simulink model "s_6dof2016a"  (R2016a)
settings: Solver=VariableStepAuto  SolverMode=SingleTasking  StartTime=0.0  StopTime=90  RelTol=1e-3
(part 1 of 2)
settings Model: Creator=Admin  LastModifiedBy=HP
settings DebuggingCC: SFUnexpectedBacktrackingDiag=error  SFNoUnconditionalDefaultTransitionDiag=error
settings GRTTargetCC: TargetLangStandard=C99 (ISO)  GeneratePreprocessorConditionals=Use local settings
settings ConfigComp: CovMetricSettings=dwe  CovHtmlReporting=off  CovSaveCumulativeToWorkspaceVar=off  CovSaveSingleToWorkspaceVar=off  CovExternalEMLEnable=on

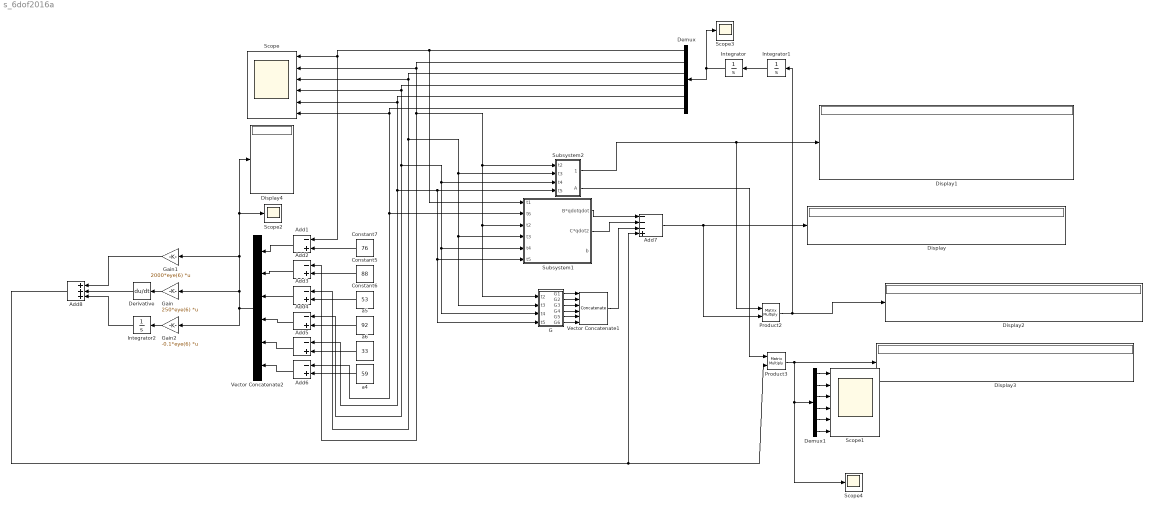
== system s_6dof2016a ==
  Add{1..6} (6 alike) : Sum  Inputs=-+
  Add7 : Sum  Inputs=---+
  Add8 : Sum  Inputs=+++
  Constant5 : Constant  Value=88
  Constant6 : Constant  Value=53
  Constant7 : Constant  Value=76
  Demux : Demux  Outputs=6
  Demux1 : Demux  Outputs=6
  Derivative : Derivative
  Display{,1..4} (5 alike) : Display
  G : Subsystem
  Gain : Gain  Gain=250*eye(6)  Multiplication=Matrix(K*u)
  Gain1 : Gain  Gain=2000*eye(6)  Multiplication=Matrix(K*u)
  Gain2 : Gain  Gain=-0.1*eye(6)  Multiplication=Matrix(K*u)
  Integrator : Integrator
  Integrator1 : Integrator
  Integrator2 : Integrator
  Product2 : Product  Multiplication=Matrix(*)
  Product3 : Product  Multiplication=Matrix(*)
  Scope : Scope  NumInputPorts=6
  Scope1 : Scope  NumInputPorts=6
  Scope2 : Scope
  Scope3 : Scope
  Scope4 : Scope
  Subsystem1 : Subsystem
  Subsystem2 : Subsystem
  Vector Concatenate1 : Concatenate  NumInputs=6  Mode=Multidimensional array
  Vector Concatenate2 : Concatenate  NumInputs=6  Mode=Multidimensional array
  a4 : Constant  Value=59
  a5 : Constant  Value=92
  a6 : Constant  Value=33
  wires:
  Demux/4 -> Scope/4, Add4/1, G/3(t4), Subsystem1/5("t4 "), Subsystem2/3(t4)
  Demux/5 -> Scope/5, Add5/1, G/4(t5), Subsystem1/6(t5), Subsystem2/4(t5)
  Demux/2 -> Scope/2, Add2/1, G/1(t2), Subsystem1/3(t2), Subsystem2/1(t2)
  Demux/3 -> Scope/3, G/2(t3), Subsystem1/4(t3), Subsystem2/2(t3), Add3/1
  Demux/1 -> Scope/1, Add1/1, Subsystem1/1(t1)
  Demux/6 -> Scope/6, Subsystem1/2(t6), Add6/1
  Constant7/1 -> Add1/2
  Constant5/1 -> Add2/2
  Constant6/1 -> Add3/2
  a5/1 -> Add4/2
  a6/1 -> Add5/2
  a4/1 -> Add6/2
  Subsystem1/1(B*qdotqdot) -> Add7/1
  Subsystem1/2(C*qdot2) -> Add7/2
  G/1(G1) -> Vector Concatenate1/1
  G/2(G2) -> Vector Concatenate1/2
  G/3(G3) -> Vector Concatenate1/3
  G/6(G6) -> Vector Concatenate1/6
  G/4(G4) -> Vector Concatenate1/4
  G/5(G5) -> Vector Concatenate1/5
  Vector Concatenate1/1 -> Add7/3
  Add7/1 -> Product2/2, Display/1
  Subsystem2/1(A inv) -> Product2/1, Display1/1
  Add2/1 -> Vector Concatenate2/2
  Add1/1 -> Vector Concatenate2/1
  Add3/1 -> Vector Concatenate2/3
  Add4/1 -> Vector Concatenate2/4
  Add5/1 -> Vector Concatenate2/5
  Add6/1 -> Vector Concatenate2/6
  Product2/1 -> Integrator1/1, Display2/1
  Integrator1/1 -> Integrator/1
  Integrator/1 -> Scope3/1, Demux/1
  Product3/1 -> Scope4/1, Demux1/1, Display3/1
  Subsystem2/2("A ") -> Product3/1
  Demux1/1 -> Scope1/1
  Demux1/2 -> Scope1/2
  Demux1/3 -> Scope1/3
  Demux1/4 -> Scope1/4
  Demux1/5 -> Scope1/5
  Demux1/6 -> Scope1/6
  Vector Concatenate2/1 -> Display4/1, Scope2/1, Gain1/1, Gain/1, Gain2/1
  Gain/1 -> Derivative/1
  Gain2/1 -> Integrator2/1
  Gain1/1 -> Add8/1
  Add8/1 -> Product3/2, Add7/4
  Derivative/1 -> Add8/2
  Integrator2/1 -> Add8/3

== system s_6dof2016a/G ==
  t2 : Inport
  t3 : Inport  Port=2
  t4 : Inport  Port=3
  t5 : Inport  Port=4
  g1 : Constant  Value=0
  g2 : Subsystem
  g3 : Subsystem
  g4 : Subsystem
  g5 : Subsystem
  g6 : Constant  Value=0
  G1 : Outport
  G2 : Outport  Port=2
  G3 : Outport  Port=3
  G4 : Outport  Port=4
  G5 : Outport  Port=5
  G6 : Outport  Port=6
  wires:
  t5/1 -> g5/2(t5), g4/2(t5)
  g3/1(g3) -> G3/1
  g5/1(g5) -> G5/1
  t3/1 -> g5/4(t3), g4/4(t3), g3/2(t3), g2/2(t3)
  t4/1 -> g5/1(t4), g4/1(t4)
  g2/1(g2) -> G2/1
  t2/1 -> g5/3(t2), g4/3(t2), g3/1(t2), g2/1(t2)
  g1/1 -> G1/1
  g4/1(g4) -> G4/1
  g6/1 -> G6/1

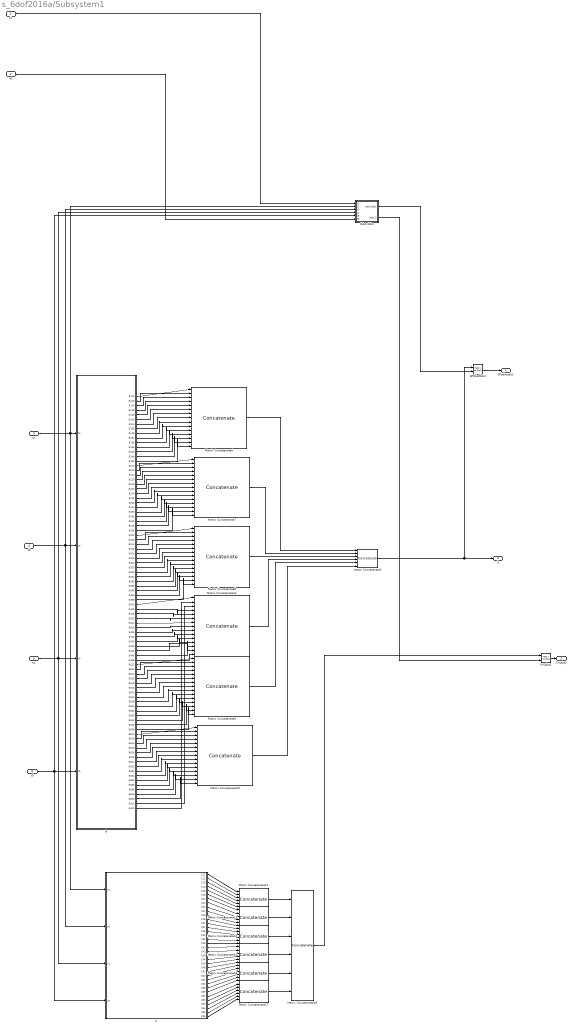
== system s_6dof2016a/Subsystem1 ==
  t1 : Inport
  t6 : Inport  Port=2
  t2 : Inport  Port=3
  t3 : Inport  Port=4
  "t4 " : Inport  Port=5
  t5 : Inport  Port=6
  B : Subsystem
  B*QdotQdot : Product  Multiplication=Matrix(*)
  C : Subsystem
  C*Qdot2 : Product  Multiplication=Matrix(*)
  Matrix Concatenate{6..11} (6 alike) : Concatenate  NumInputs=15  Mode=Multidimensional array  ConcatenateDimension=2
  Matrix Concatenate{12..17} (6 alike) : Concatenate  NumInputs=6  Mode=Multidimensional array  ConcatenateDimension=2
  Matrix Concatenate18 : Concatenate  NumInputs=6  Mode=Multidimensional array
  Qdot,Qdot : Subsystem
  Vector Concatenate1 : Concatenate  NumInputs=6  Mode=Multidimensional array
  B*qdotqdot : Outport
  C*qdot2 : Outport  Port=2
  "b " : Outport  Port=3
  wires:
  C/29(C55) -> Matrix Concatenate16/5
  C/31(C61) -> Matrix Concatenate17/1
  B/15(B156) -> Matrix Concatenate6/15
  C/25(C51) -> Matrix Concatenate16/1
  B/47(B415) -> Matrix Concatenate11/4
  C/24(C46) -> Matrix Concatenate15/6
  B/22(B224) -> Matrix Concatenate7/7
  "t4 "/1 -> C/3(t4), Qdot,Qdot/4(t4), B/3(t4)
  B/36(B323) -> Matrix Concatenate8/6
  C/30(C56) -> Matrix Concatenate16/6
  B*QdotQdot/1 -> B*qdotqdot/1
  B/37(B324) -> Matrix Concatenate8/7
  t5/1 -> Qdot,Qdot/5(t5), C/4(t5), B/4(t5)
  B/17(B213) -> Matrix Concatenate7/2
  C/10(C24) -> Matrix Concatenate13/4
  C/28(C54) -> Matrix Concatenate16/4
  B/10(B134) -> Matrix Concatenate6/10
  C/33(C63) -> Matrix Concatenate17/3
  Qdot,Qdot/2(qdot,2) -> C*Qdot2/2
  B/26(B235) -> Matrix Concatenate7/11
  C/7(C21) -> Matrix Concatenate13/1
  C/20(C42) -> Matrix Concatenate15/2
  B/67(B526) -> Matrix Concatenate9/9
  C/23(C45) -> Matrix Concatenate15/5
  B/7(B124) -> Matrix Concatenate6/7
  B/84(B635) -> Matrix Concatenate10/11
  C/11(C25) -> Matrix Concatenate13/5
  B/14(B146) -> Matrix Concatenate6/14
  C/19(C41) -> Matrix Concatenate15/1
  C/26(C52) -> Matrix Concatenate16/2
  B/45(B356) -> Matrix Concatenate8/15
  B/24(B226) -> Matrix Concatenate7/9
  C/35(C65) -> Matrix Concatenate17/5
  B/59(B512) -> Matrix Concatenate9/1
  C/6(C16) -> Matrix Concatenate12/6
  B/23(B225) -> Matrix Concatenate7/8
  C/21(C43) -> Matrix Concatenate15/3
  B/13(B145) -> Matrix Concatenate6/13
  C/36(C66) -> Matrix Concatenate17/6
  t2/1 -> Qdot,Qdot/2(t2), C/1(t2), B/1(t2)
  C/32(C62) -> Matrix Concatenate17/2
  B/63(B516) -> Matrix Concatenate9/5
  t3/1 -> Qdot,Qdot/3(t3), C/2(t3), B/2(t3)
  Matrix Concatenate12/1 -> Matrix Concatenate18/1
  B/65(B524) -> Matrix Concatenate9/7
  C/8(C22) -> Matrix Concatenate13/2
  B/6(B123) -> Matrix Concatenate6/6
  C/13(C31) -> Matrix Concatenate14/1
  B/61(B514) -> Matrix Concatenate9/3
  Matrix Concatenate18/1 -> C*Qdot2/1
  C/9(C23) -> Matrix Concatenate13/3
  C/12(C26) -> Matrix Concatenate13/6
  B/78(B616) -> Matrix Concatenate10/5
  B/4(B115) -> Matrix Concatenate6/4
  B/35(B316) -> Matrix Concatenate8/5
  C/16(C34) -> Matrix Concatenate14/4
  C/14(C32) -> Matrix Concatenate14/2
  B/66(B525) -> Matrix Concatenate9/8
  C/18(C36) -> Matrix Concatenate14/6
  B/32(B313) -> Matrix Concatenate8/2
  C/17(C35) -> Matrix Concatenate14/5
  B/2(B113) -> Matrix Concatenate6/2
  B/25(B234) -> Matrix Concatenate7/10
  B/11(B135) -> Matrix Concatenate6/11
  B/18(B214) -> Matrix Concatenate7/3
  B/77(B615) -> Matrix Concatenate10/4
  B/5(B116) -> Matrix Concatenate6/5
  B/64(B523) -> Matrix Concatenate9/6
  t1/1 -> Qdot,Qdot/1(t1)
  B/3(B114) -> Matrix Concatenate6/3
  B/27(B236) -> Matrix Concatenate7/12
  B/28(B245) -> Matrix Concatenate7/13
  B/30(B256) -> Matrix Concatenate7/15
  B/51(B425) -> Matrix Concatenate11/8
  B/40(B334) -> Matrix Concatenate8/10
  B/60(B513) -> Matrix Concatenate9/2
  B/70(B536) -> Matrix Concatenate9/12
  B/74(B612) -> Matrix Concatenate10/1
  B/75(B613) -> Matrix Concatenate10/2
  B/79(B623) -> Matrix Concatenate10/6
  B/80(B624) -> Matrix Concatenate10/7
  B/21(B223) -> Matrix Concatenate7/6
  t6/1 -> Qdot,Qdot/6(t6)
  B/31(B312) -> Matrix Concatenate8/1
  B/42(B336) -> Matrix Concatenate8/12
  B/81(B625) -> Matrix Concatenate10/8
  B/9(B126) -> Matrix Concatenate6/9
  B/68(B534) -> Matrix Concatenate9/10
  B/29(B246) -> Matrix Concatenate7/14
  B/38(B325) -> Matrix Concatenate8/8
  B/52(B426) -> Matrix Concatenate11/9
  B/82(B626) -> Matrix Concatenate10/9
  B/86(B645) -> Matrix Concatenate10/13
  B/43(B345) -> Matrix Concatenate8/13
  B/71(B545) -> Matrix Concatenate9/13
  B/87(B646) -> Matrix Concatenate10/14
  B/46(B412) -> Matrix Concatenate11/1
  B/83(B634) -> Matrix Concatenate10/10
  B/89(B414) -> Matrix Concatenate11/3
  B/69(B535) -> Matrix Concatenate9/11
  B/33(B314) -> Matrix Concatenate8/3
  B/20(B216) -> Matrix Concatenate7/5
  B/90(B413) -> Matrix Concatenate11/2
  B/76(B614) -> Matrix Concatenate10/3
  B/50(B424) -> Matrix Concatenate11/7
  B/19(B215) -> Matrix Concatenate7/4
  B/62(B515) -> Matrix Concatenate9/4
  B/57(B446) -> Matrix Concatenate11/14
  Matrix Concatenate7/1 -> Vector Concatenate1/2
  B/48(B416) -> Matrix Concatenate11/5
  B/34(B315) -> Matrix Concatenate8/4
  B/1(B112) -> Matrix Concatenate6/1
  B/53(B434) -> Matrix Concatenate11/10
  B/54(B435) -> Matrix Concatenate11/11
  Matrix Concatenate14/1 -> Matrix Concatenate18/3
  B/73(B556) -> Matrix Concatenate9/15
  Matrix Concatenate8/1 -> Vector Concatenate1/3
  C/1(C11) -> Matrix Concatenate12/1
  B/85(B636) -> Matrix Concatenate10/12
  Matrix Concatenate9/1 -> Vector Concatenate1/5
  B/39(B326) -> Matrix Concatenate8/9
  B/49(B423) -> Matrix Concatenate11/6
  Matrix Concatenate11/1 -> Vector Concatenate1/4
  B/55(B436) -> Matrix Concatenate11/12
  B/41(B335) -> Matrix Concatenate8/11
  B/16(B212) -> Matrix Concatenate7/1
  Matrix Concatenate10/1 -> Vector Concatenate1/6
  C/34(C64) -> Matrix Concatenate17/4
  B/56(B445) -> Matrix Concatenate11/13
  B/44(B346) -> Matrix Concatenate8/14
  B/88(B656) -> Matrix Concatenate10/15
  Qdot,Qdot/1(qdot,qdot) -> B*QdotQdot/2
  B/72(B546) -> Matrix Concatenate9/14
  B/12(B136) -> Matrix Concatenate6/12
  B/58(B456) -> Matrix Concatenate11/15
  Matrix Concatenate6/1 -> Vector Concatenate1/1
  B/8(B125) -> Matrix Concatenate6/8
  Vector Concatenate1/1 -> "b "/1, B*QdotQdot/1
  C/22(C44) -> Matrix Concatenate15/4
  C/15(C33) -> Matrix Concatenate14/3
  C/27(C53) -> Matrix Concatenate16/3
  Matrix Concatenate17/1 -> Matrix Concatenate18/6
  Matrix Concatenate16/1 -> Matrix Concatenate18/5
  Matrix Concatenate13/1 -> Matrix Concatenate18/2
  Matrix Concatenate15/1 -> Matrix Concatenate18/4
  C/3(C13) -> Matrix Concatenate12/3
  C/2(C12) -> Matrix Concatenate12/2
  C/4(C14) -> Matrix Concatenate12/4
  C/5(C15) -> Matrix Concatenate12/5
  C*Qdot2/1 -> C*qdot2/1

== system s_6dof2016a/Subsystem2 ==
  t2 : Inport
  t3 : Inport  Port=2
  t4 : Inport  Port=3
  t5 : Inport  Port=4
  Divide : Product  Inputs=/  Multiplication=Matrix(*)
  Matrix Concatenate{,1..5} (6 alike) : Concatenate  NumInputs=6  Mode=Multidimensional array  ConcatenateDimension=2
  Subsystem : Subsystem
  Vector Concatenate : Concatenate  NumInputs=6  Mode=Multidimensional array
  A inv : Outport
  "A " : Outport  Port=2
  wires:
  Subsystem/5(A15) -> Matrix Concatenate/5
  Subsystem/13(A31) -> Matrix Concatenate2/1
  Subsystem/12(A26) -> Matrix Concatenate1/6
  Subsystem/36(A66) -> Matrix Concatenate5/6
  Subsystem/1(A11) -> Matrix Concatenate/1
  Subsystem/24(A46) -> Matrix Concatenate3/6
  Subsystem/3(A13) -> Matrix Concatenate/3
  Subsystem/2(A12) -> Matrix Concatenate/2
  Subsystem/26(A52) -> Matrix Concatenate4/2
  Subsystem/28(A54) -> Matrix Concatenate4/4
  t5/1 -> Subsystem/4("t5 ")
  Subsystem/10(A24) -> Matrix Concatenate1/4
  Subsystem/9(A23) -> Matrix Concatenate1/3
  Subsystem/15(A33) -> Matrix Concatenate2/3
  Subsystem/11(A25) -> Matrix Concatenate1/5
  Subsystem/34(A64) -> Matrix Concatenate5/4
  Subsystem/18(A36) -> Matrix Concatenate2/6
  Matrix Concatenate4/1 -> Vector Concatenate/5
  Subsystem/19(A41) -> Matrix Concatenate3/1
  Subsystem/20(A42) -> Matrix Concatenate3/2
  Subsystem/23(A45) -> Matrix Concatenate3/5
  Subsystem/29(A55) -> Matrix Concatenate4/5
  Subsystem/30(A56) -> Matrix Concatenate4/6
  Subsystem/7(A21) -> Matrix Concatenate1/1
  t2/1 -> Subsystem/1(t2)
  Subsystem/33(A63) -> Matrix Concatenate5/3
  Subsystem/35(A65) -> Matrix Concatenate5/5
  Matrix Concatenate/1 -> Vector Concatenate/1
  Matrix Concatenate1/1 -> Vector Concatenate/2
  Matrix Concatenate2/1 -> Vector Concatenate/3
  Subsystem/21(A43) -> Matrix Concatenate3/3
  Subsystem/22(A44) -> Matrix Concatenate3/4
  Subsystem/25(A51) -> Matrix Concatenate4/1
  Subsystem/8(A22) -> Matrix Concatenate1/2
  Subsystem/4(A14) -> Matrix Concatenate/4
  Subsystem/6(A16) -> Matrix Concatenate/6
  Subsystem/31(A61) -> Matrix Concatenate5/1
  Subsystem/27(A53) -> Matrix Concatenate4/3
  Subsystem/17(A35) -> Matrix Concatenate2/5
  Matrix Concatenate5/1 -> Vector Concatenate/6
  Subsystem/14(A32) -> Matrix Concatenate2/2
  Subsystem/32(A62) -> Matrix Concatenate5/2
  t4/1 -> Subsystem/3(t4)
  Subsystem/16(A34) -> Matrix Concatenate2/4
  Matrix Concatenate3/1 -> Vector Concatenate/4
  t3/1 -> Subsystem/2(t3)
  Vector Concatenate/1 -> "A "/1, Divide/1
  Divide/1 -> A inv/1

== system s_6dof2016a/G/g2 ==
  t2 : Inport
  t3 : Inport  Port=2
  Add1 : Sum
  Add2 : Sum  Inputs=+++
  Product2 : Product
  Product3 : Product
  Product4 : Product
  Trigonometric Function1 : Trigonometry  Operator=cos
  Trigonometric Function4 : Trigonometry
  Trigonometric Function6 : Trigonometry
  c : Constant  Value=-37.2
  c2 : Constant  Value=-8.4
  c3 : Constant  Value=1.02
  g2 : Outport
  wires:
  c2/1 -> Product3/1
  t2/1 -> Trigonometric Function6/1, Add1/1, Trigonometric Function1/1
  Product4/1 -> Add2/3
  Product2/1 -> Add2/1
  Trigonometric Function6/1 -> Product4/2
  c3/1 -> Product4/1
  Add1/1 -> Trigonometric Function4/1
  Add2/1 -> g2/1
  Trigonometric Function4/1 -> Product3/2
  Product3/1 -> Add2/2
  Trigonometric Function1/1 -> Product2/2
  c/1 -> Product2/1
  t3/1 -> Add1/2

== system s_6dof2016a/G/g3 ==
  t2 : Inport
  t3 : Inport  Port=2
  Add1 : Sum
  Add2 : Sum
  Product2 : Product
  Product3 : Product
  Trigonometric Function1 : Trigonometry
  Trigonometric Function4 : Trigonometry  Operator=cos
  c2 : Constant  Value=-8.4
  c3 : Constant  Value=0.25
  g3 : Outport
  wires:
  Product2/1 -> Add2/1
  Trigonometric Function1/1 -> Product2/2
  Add1/1 -> Trigonometric Function4/1, Trigonometric Function1/1
  c2/1 -> Product2/1
  Product3/1 -> Add2/2
  t3/1 -> Add1/2
  c3/1 -> Product3/1
  t2/1 -> Add1/1
  Trigonometric Function4/1 -> Product3/2
  Add2/1 -> g3/1

== system s_6dof2016a/G/g4 ==
  t4 : Inport
  t5 : Inport  Port=2
  t2 : Inport  Port=3
  t3 : Inport  Port=4
  Add1 : Sum
  Product2 : Product  Inputs=4
  Trigonometric Function1 : Trigonometry
  Trigonometric Function4 : Trigonometry
  Trigonometric Function6 : Trigonometry
  c2 : Constant  Value=0.028
  g4 : Outport
  wires:
  t4/1 -> Trigonometric Function4/1
  Trigonometric Function4/1 -> Product2/3
  Product2/1 -> g4/1
  c2/1 -> Product2/1
  t5/1 -> Trigonometric Function6/1
  t2/1 -> Add1/1
  Trigonometric Function1/1 -> Product2/2
  Add1/1 -> Trigonometric Function1/1
  Trigonometric Function6/1 -> Product2/4
  t3/1 -> Add1/2

== system s_6dof2016a/G/g5 ==
  t4 : Inport
  t5 : Inport  Port=2
  t2 : Inport  Port=3
  t3 : Inport  Port=4
  Add1 : Sum
  Add2 : Sum
  Product2 : Product
  Product3 : Product  Inputs=3
  Product4 : Product
  Trigonometric Function1 : Trigonometry  Operator=cos
  Trigonometric Function4 : Trigonometry
  Trigonometric Function6 : Trigonometry
  Trigonometric Function7 : Trigonometry  Operator=cos
  Trigonometric Function8 : Trigonometry  Operator=cos
  c2 : Constant  Value=-0.028
  g5 : Outport
  wires:
  Add1/1 -> Trigonometric Function6/1, Trigonometric Function1/1
  c2/1 -> Product4/1
  Trigonometric Function1/1 -> Product2/1
  t5/1 -> Trigonometric Function8/1, Trigonometric Function4/1
  Trigonometric Function7/1 -> Product3/2
  Trigonometric Function6/1 -> Product3/1
  Trigonometric Function8/1 -> Product3/3
  Trigonometric Function4/1 -> Product2/2
  t2/1 -> Add1/1
  Product2/1 -> Add2/1
  Add2/1 -> Product4/2
  Product3/1 -> Add2/2
  t3/1 -> Add1/2
  t4/1 -> Trigonometric Function7/1
  Product4/1 -> g5/1

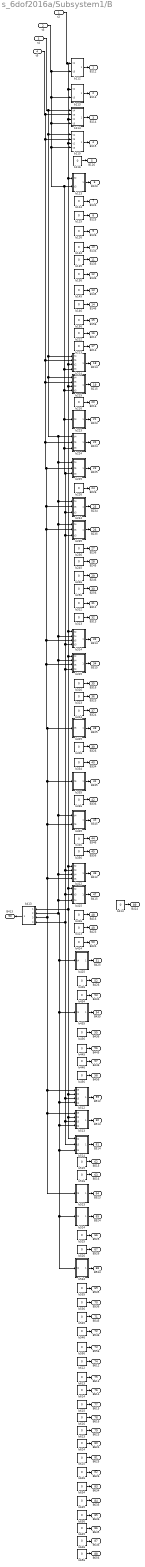
== system s_6dof2016a/Subsystem1/B ==
  t2 : Inport
  t3 : Inport  Port=2
  t4 : Inport  Port=3
  t5 : Inport  Port=4
  b112 : Subsystem
  b113 : Subsystem
  b114 : Subsystem
  b115 : Subsystem
  b{116,124..126,134..136,145..146,156,212..213,216,226,236,245..246,256,312..313,316,323..324,326,334,336,346,356,414,416,423..424,426,434,436,445..446,456,515..516,525..526,535..536,545..546,556,612..616,623..626,634..636,645..646,656} (62 alike) : Constant  Value=0
  b123 : Subsystem
  b214 : Subsystem
  b215 : Subsystem
  b223 : Subsystem
  b224 : Subsystem
  b225 : Subsystem
  b234 : Subsystem
  b235 : Subsystem
  b314 : Subsystem
  b315 : Subsystem
  b325 : Subsystem
  b335 : Subsystem
  b345 : Subsystem
  b412 : Subsystem
  b413 : Subsystem
  b415 : Subsystem
  b425 : Subsystem
  b435 : Subsystem
  b512 : Subsystem
  b513 : Subsystem
  b514 : Subsystem
  b523 : Subsystem
  b524 : Subsystem
  b534 : Subsystem
  B112 : Outport
  B113 : Outport  Port=2
  B114 : Outport  Port=3
  B115 : Outport  Port=4
  B116 : Outport  Port=5
  B123 : Outport  Port=6
  B124 : Outport  Port=7
  B125 : Outport  Port=8
  B126 : Outport  Port=9
  B134 : Outport  Port=10
  B135 : Outport  Port=11
  B136 : Outport  Port=12
  B145 : Outport  Port=13
  B146 : Outport  Port=14
  B156 : Outport  Port=15
  B212 : Outport  Port=16
  B213 : Outport  Port=17
  B214 : Outport  Port=18
  B215 : Outport  Port=19
  B216 : Outport  Port=20
  B223 : Outport  Port=21
  B224 : Outport  Port=22
  B225 : Outport  Port=23
  B226 : Outport  Port=24
  B234 : Outport  Port=25
  B235 : Outport  Port=26
  B236 : Outport  Port=27
  B245 : Outport  Port=28
  B246 : Outport  Port=29
  B256 : Outport  Port=30
  B312 : Outport  Port=31
  B313 : Outport  Port=32
  B314 : Outport  Port=33
  B315 : Outport  Port=34
  B316 : Outport  Port=35
  B323 : Outport  Port=36
  B324 : Outport  Port=37
  B325 : Outport  Port=38
  B326 : Outport  Port=39
  B334 : Outport  Port=40
  B335 : Outport  Port=41
  B336 : Outport  Port=42
  B345 : Outport  Port=43
  B346 : Outport  Port=44
  B356 : Outport  Port=45
  B412 : Outport  Port=46
  B415 : Outport  Port=47
  B416 : Outport  Port=48
  B423 : Outport  Port=49
  B424 : Outport  Port=50
  B425 : Outport  Port=51
  B426 : Outport  Port=52
  B434 : Outport  Port=53
  B435 : Outport  Port=54
  B436 : Outport  Port=55
  B445 : Outport  Port=56
  B446 : Outport  Port=57
  B456 : Outport  Port=58
  B512 : Outport  Port=59
  B513 : Outport  Port=60
  B514 : Outport  Port=61
  B515 : Outport  Port=62
  B516 : Outport  Port=63
  B523 : Outport  Port=64
  B524 : Outport  Port=65
  B525 : Outport  Port=66
  B526 : Outport  Port=67
  B534 : Outport  Port=68
  B535 : Outport  Port=69
  B536 : Outport  Port=70
  B545 : Outport  Port=71
  B546 : Outport  Port=72
  B556 : Outport  Port=73
  B612 : Outport  Port=74
  B613 : Outport  Port=75
  B614 : Outport  Port=76
  B615 : Outport  Port=77
  B616 : Outport  Port=78
  B623 : Outport  Port=79
  B624 : Outport  Port=80
  B625 : Outport  Port=81
  B626 : Outport  Port=82
  B634 : Outport  Port=83
  B635 : Outport  Port=84
  B636 : Outport  Port=85
  B645 : Outport  Port=86
  B646 : Outport  Port=87
  B656 : Outport  Port=88
  B414 : Outport  Port=89
  B413 : Outport  Port=90
  wires:
  b514/1(b514) -> B514/1
  b313/1 -> B313/1
  t4/1 -> b534/1(t4), b524/1(t4), b514/3(t4), b513/4(t4), b512/4(t4), b435/1(t4), b425/1(t4), b413/2(In2), b415/3(t4), b412/3(t4), b345/1(t4), b315/2(t4), b314/2(t4), b235/1(t4), b234/1(t4), b225/1(t4), b224/1(t4), b215/1(t4), b214/1(t4), b115/1(t4), b114/1(t4)
  b446/1 -> B446/1
  t3/1 -> b113/2(t3), b115/4(t3), b514/2(t3), b513/3(t3), b512/3(t3), b413/4(In4), b415/2(t3), b412/2(t3), b315/4(t3), b314/4(t3), b235/3(t3), b234/3(t3), b225/3(t3), b224/3(t3), b223/1(t3), b215/4(t3), b214/4(t3), b123/2("t3 "), b114/4(t3), b112/2(t3)
  t2/1 -> b514/1(t2), b513/2(t2), b512/2(t2), b413/1(In1), b415/1(t2), b412/1(t2), b315/1(t2), b314/1(t2), b215/3(t2), b214/3(t2), b123/1(t2), b115/3(t2), b114/3(t2), b113/1(t2), b112/1(t2)
  b625/1 -> B625/1
  t5/1 -> b523/1(t5), b513/1(t5), b512/1(t5), b413/3(In3), b412/4(t5), b345/2(t5), b335/1(t5), b325/1(t5), b315/3(t5), b314/3(t5), b235/2(t5), b234/2(t5), b225/2(t5), b224/2(t5), b215/2(t5), b214/2(t5), b115/2(t5), b114/2(t5)
  b312/1 -> B312/1
  b326/1 -> B326/1
  b345/1(b345) -> B345/1
  b636/1 -> B636/1
  b656/1 -> B656/1
  b145/1 -> B145/1
  b136/1 -> B136/1
  b115/1(b115) -> B115/1
  b546/1 -> B546/1
  b526/1 -> B526/1
  b445/1 -> B445/1
  b626/1 -> B626/1
  b545/1 -> B545/1
  b515/1 -> B515/1
  b325/1(b325) -> B325/1
  b134/1 -> B134/1
  b135/1 -> B135/1
  b246/1 -> B246/1
  b215/1(b215) -> B215/1
  b123/1(b123) -> B123/1
  b126/1 -> B126/1
  b225/1(b225) -> B225/1
  b623/1 -> B623/1
  b356/1 -> B356/1
  b523/1(b523) -> B523/1
  b234/1(b224) -> B234/1
  b114/1(b114) -> B114/1
  b534/1(b524) -> B534/1
  b113/1(b113) -> B113/1
  b335/1(b325) -> B335/1
  b613/1 -> B613/1
  b646/1 -> B646/1
  b245/1 -> B245/1
  b624/1 -> B624/1
  b146/1 -> B146/1
  b223/1(b223) -> B223/1
  b124/1 -> B124/1
  b535/1 -> B535/1
  b616/1 -> B616/1
  b116/1 -> B116/1
  b212/1 -> B212/1
  b436/1 -> B436/1
  b112/1(b112) -> B112/1
  b213/1 -> B213/1
  b156/1 -> B156/1
  b512/1(b512) -> B512/1
  b214/1(b214) -> B214/1
  b645/1 -> B645/1
  b315/1(b315) -> B315/1
  b415/1(b415) -> B415/1
  b536/1 -> B536/1
  b425/1(b425) -> B425/1
  b324/1 -> B324/1
  b612/1 -> B612/1
  b635/1 -> B635/1
  b634/1 -> B634/1
  b615/1 -> B615/1
  b516/1 -> B516/1
  b423/1 -> B423/1
  b424/1 -> B424/1
  b316/1 -> B316/1
  b336/1 -> B336/1
  b334/1 -> B334/1
  b426/1 -> B426/1
  b256/1 -> B256/1
  b235/1(b225) -> B235/1
  b226/1 -> B226/1
  b416/1 -> B416/1
  b224/1(b224) -> B224/1
  b216/1 -> B216/1
  b456/1 -> B456/1
  b236/1 -> B236/1
  b525/1 -> B525/1
  b513/1(b513) -> B513/1
  b614/1 -> B614/1
  b434/1 -> B434/1
  b346/1 -> B346/1
  b556/1 -> B556/1
  b435/1(b425) -> B435/1
  b412/1(b412) -> B412/1
  b524/1(b524) -> B524/1
  b125/1 -> B125/1
  b314/1(b314) -> B314/1
  b323/1 -> B323/1
  b414/1 -> B414/1
  b413/1(b413) -> B413/1

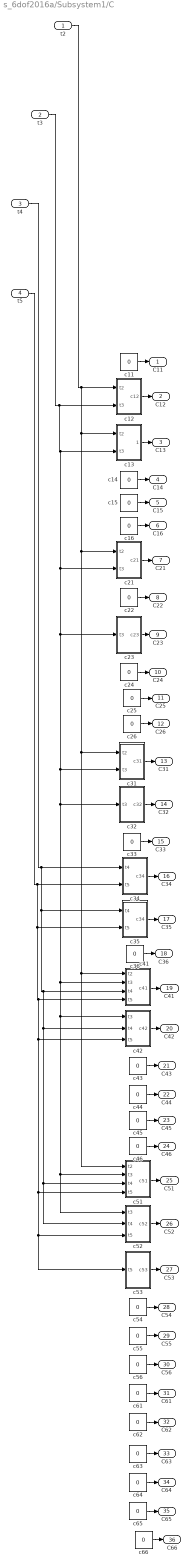
== system s_6dof2016a/Subsystem1/C ==
  t2 : Inport
  t3 : Inport  Port=2
  t4 : Inport  Port=3
  t5 : Inport  Port=4
  c{11,14..16,22,24..26,33,36,43..46,54..56,61..66} (23 alike) : Constant  Value=0
  c12 : Subsystem
  c13 : Subsystem
  c21 : Subsystem
  c23 : Subsystem
  c31 : Subsystem
  c32 : Subsystem
  c34 : Subsystem
  c35 : Subsystem
  c41 : Subsystem
  c42 : Subsystem
  c51 : Subsystem
  c52 : Subsystem
  c53 : Subsystem
  C11 : Outport
  C12 : Outport  Port=2
  C13 : Outport  Port=3
  C14 : Outport  Port=4
  C15 : Outport  Port=5
  C16 : Outport  Port=6
  C21 : Outport  Port=7
  C22 : Outport  Port=8
  C23 : Outport  Port=9
  C24 : Outport  Port=10
  C25 : Outport  Port=11
  C26 : Outport  Port=12
  C31 : Outport  Port=13
  C32 : Outport  Port=14
  C33 : Outport  Port=15
  C34 : Outport  Port=16
  C35 : Outport  Port=17
  C36 : Outport  Port=18
  C41 : Outport  Port=19
  C42 : Outport  Port=20
  C43 : Outport  Port=21
  C44 : Outport  Port=22
  C45 : Outport  Port=23
  C46 : Outport  Port=24
  C51 : Outport  Port=25
  C52 : Outport  Port=26
  C53 : Outport  Port=27
  C54 : Outport  Port=28
  C55 : Outport  Port=29
  C56 : Outport  Port=30
  C61 : Outport  Port=31
  C62 : Outport  Port=32
  C63 : Outport  Port=33
  C64 : Outport  Port=34
  C65 : Outport  Port=35
  C66 : Outport  Port=36
  wires:
  c64/1 -> C64/1
  c35/1(c34) -> C35/1
  c42/1(c42) -> C42/1
  c14/1 -> C14/1
  t2/1 -> c51/1(t2), c41/1(t2), c31/1(t2), c21/1(t2), c13/1(t2), c12/1(t2)
  c24/1 -> C24/1
  t5/1 -> c53/1(t5), c52/3(t5), c51/4(t5), c42/3(t5), c41/4(t5), c35/2(t5), c34/2(t5)
  t3/1 -> c52/1(t3), c51/2(t3), c42/1(t3), c41/2(t3), c32/1(t3), c31/2(t3), c23/1(t3), c21/2(t3), c13/2("t3 "), c12/2(t3)
  t4/1 -> c52/2(t4), c51/3(t4), c42/2(t4), c41/3(t4), c35/1(t4), c34/1(t4)
  c54/1 -> C54/1
  c62/1 -> C62/1
  c25/1 -> C25/1
  c53/1(c53) -> C53/1
  c45/1 -> C45/1
  c61/1 -> C61/1
  c44/1 -> C44/1
  c21/1(c21) -> C21/1
  c31/1(c31) -> C31/1
  c55/1 -> C55/1
  c56/1 -> C56/1
  c63/1 -> C63/1
  c52/1(c52) -> C52/1
  c34/1(c34) -> C34/1
  c41/1(c41) -> C41/1
  c66/1 -> C66/1
  c32/1(c32) -> C32/1
  c46/1 -> C46/1
  c16/1 -> C16/1
  c65/1 -> C65/1
  c36/1 -> C36/1
  c26/1 -> C26/1
  c11/1 -> C11/1
  c15/1 -> C15/1
  c43/1 -> C43/1
  c33/1 -> C33/1
  c23/1(c23) -> C23/1
  c22/1 -> C22/1
  c13/1(b123) -> C13/1
  c51/1(c51) -> C51/1
  c12/1(c12) -> C12/1

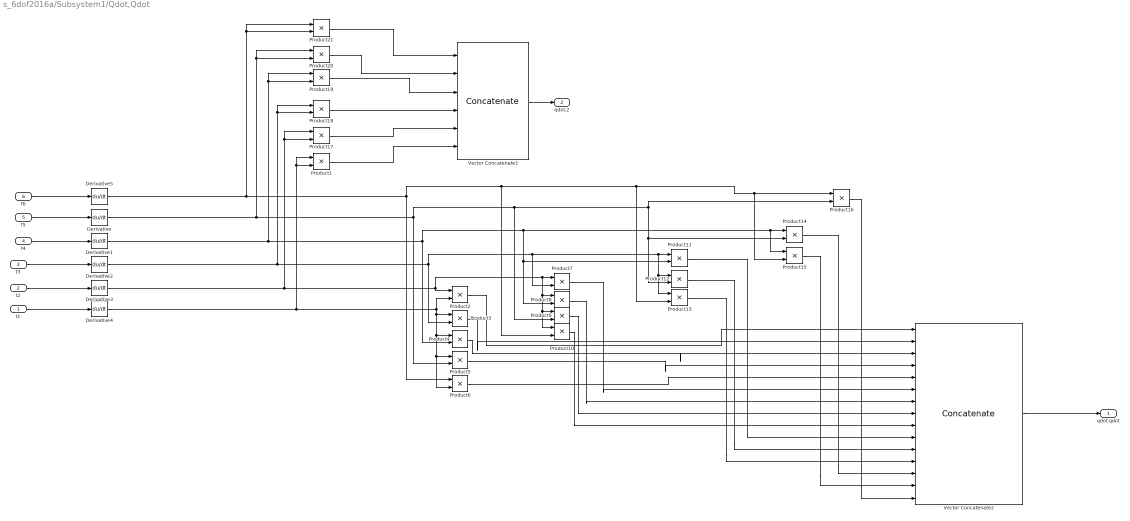
== system s_6dof2016a/Subsystem1/Qdot,Qdot ==
  t1 : Inport
  t2 : Inport  Port=2
  t3 : Inport  Port=3
  t4 : Inport  Port=4
  t5 : Inport  Port=5
  t6 : Inport  Port=6
  Derivative{,1..5} (6 alike) : Derivative
  Product{1..21} (21 alike) : Product
  Vector Concatenate1 : Concatenate  NumInputs=6
  Vector Concatenate2 : Concatenate  NumInputs=15
  qdot,qdot : Outport
  qdot,2 : Outport  Port=2
  wires:
  Derivative2/1 -> Product18/1, Product18/2, Product13/1, Product12/1, Product11/1, Product7/2, Product3/2
  Derivative/1 -> Product20/1, Product20/2, Product16/2, Product14/2, Product12/2, Product9/2, Product5/2
  Product12/1 -> Vector Concatenate2/11
  Product8/1 -> Vector Concatenate2/7
  Derivative5/1 -> Product21/1, Product21/2, Product15/2, Product16/1, Product13/2, Product10/2, Product6/1
  Product10/1 -> Vector Concatenate2/9
  Derivative4/1 -> Product2/2, Product6/2, Product5/1, Product4/1, Product3/1, Product1/1, Product1/2
  Product7/1 -> Vector Concatenate2/6
  Product14/1 -> Vector Concatenate2/13
  Derivative1/1 -> Product19/1, Product19/2, Product15/1, Product14/1, Product11/2, Product8/2, Product4/2
  Derivative3/1 -> Product17/1, Product17/2, Product10/1, Product9/1, Product8/1, Product7/1, Product2/1
  Product4/1 -> Vector Concatenate2/3
  Product13/1 -> Vector Concatenate2/12
  Product3/1 -> Vector Concatenate2/2
  Product6/1 -> Vector Concatenate2/5
  Product5/1 -> Vector Concatenate2/4
  Product11/1 -> Vector Concatenate2/10
  Product2/1 -> Vector Concatenate2/1
  Product9/1 -> Vector Concatenate2/8
  Product16/1 -> Vector Concatenate2/15
  Product15/1 -> Vector Concatenate2/14
  t1/1 -> Derivative4/1
  Vector Concatenate2/1 -> qdot,qdot/1
  t2/1 -> Derivative3/1
  t6/1 -> Derivative5/1
  t5/1 -> Derivative/1
  t3/1 -> Derivative2/1
  t4/1 -> Derivative1/1
  Product18/1 -> Vector Concatenate1/4
  Product21/1 -> Vector Concatenate1/1
  Product20/1 -> Vector Concatenate1/2
  Product19/1 -> Vector Concatenate1/3
  Product17/1 -> Vector Concatenate1/5
  Product1/1 -> Vector Concatenate1/6
  Vector Concatenate1/1 -> qdot,2/1

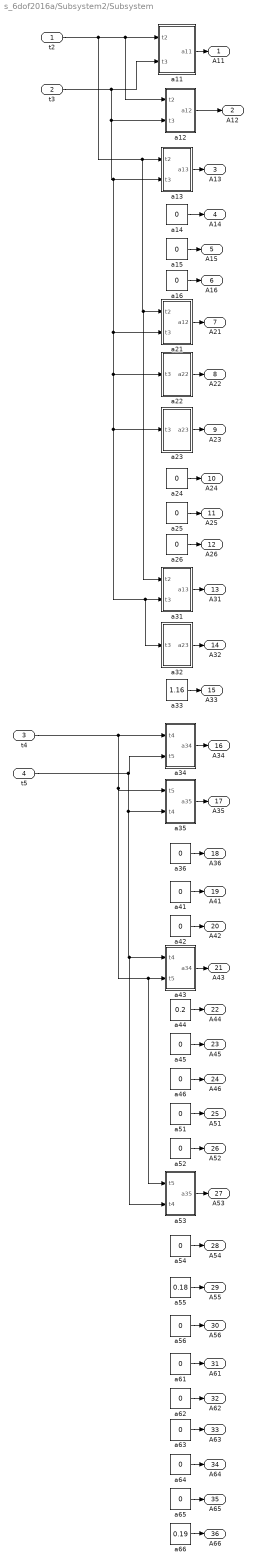
== system s_6dof2016a/Subsystem2/Subsystem ==
  t2 : Inport
  t3 : Inport  Port=2
  t4 : Inport  Port=3
  "t5 " : Inport  Port=4
  a11 : Subsystem
  a12 : Subsystem
  a13 : Subsystem
  "a14 " : Constant  Value=0
  "a15 " : Constant  Value=0
  a{16,25..26,36,41..42,46,51..52,54,56,61..64} (15 alike) : Constant  Value=0
  a21 : Subsystem
  a22 : Subsystem
  a23 : Subsystem
  "a24 " : Constant  Value=0
  a31 : Subsystem
  a32 : Subsystem
  a33 : Constant  Value=1.16
  a34 : Subsystem
  a35 : Subsystem
  a43 : Subsystem
  a44 : Constant  Value=0.2
  "a45 " : Constant  Value=0
  a53 : Subsystem
  a55 : Constant  Value=0.18
  "a65 " : Constant  Value=0
  a66 : Constant  Value=0.19
  A11 : Outport
  A12 : Outport  Port=2
  A13 : Outport  Port=3
  A14 : Outport  Port=4
  A15 : Outport  Port=5
  A16 : Outport  Port=6
  A21 : Outport  Port=7
  A22 : Outport  Port=8
  A23 : Outport  Port=9
  A24 : Outport  Port=10
  A25 : Outport  Port=11
  A26 : Outport  Port=12
  A31 : Outport  Port=13
  A32 : Outport  Port=14
  A33 : Outport  Port=15
  A34 : Outport  Port=16
  A35 : Outport  Port=17
  A36 : Outport  Port=18
  A41 : Outport  Port=19
  A42 : Outport  Port=20
  A43 : Outport  Port=21
  A44 : Outport  Port=22
  A45 : Outport  Port=23
  A46 : Outport  Port=24
  A51 : Outport  Port=25
  A52 : Outport  Port=26
  A53 : Outport  Port=27
  A54 : Outport  Port=28
  A55 : Outport  Port=29
  A56 : Outport  Port=30
  A61 : Outport  Port=31
  A62 : Outport  Port=32
  A63 : Outport  Port=33
  A64 : Outport  Port=34
  A65 : Outport  Port=35
  A66 : Outport  Port=36
  wires:
  a52/1 -> A52/1
  t3/1 -> a22/1(t3), a32/1("t3 "), a31/2("t3 "), a23/1("t3 "), a21/2(t3), a13/2("t3 "), a12/2(t3), a11/2(t3)
  t2/1 -> a31/1("t2 "), a21/1(t2), a13/1("t2 "), a12/1(t2), a11/1(t2)
  a31/1("a13 ") -> A31/1
  a63/1 -> A63/1
  "a24 "/1 -> A24/1
  a11/1(a11) -> A11/1
  a54/1 -> A54/1
  "t5 "/1 -> a53/2("t4 "), a43/1(t4), a35/2("t4 "), a34/2(t5)
  a13/1("a13 ") -> A13/1
  t4/1 -> a43/2(t5), a53/1(t5), a35/1(t5), a34/1(t4)
  a53/1(a35) -> A53/1
  a62/1 -> A62/1
  "a14 "/1 -> A14/1
  a44/1 -> A44/1
  a41/1 -> A41/1
  a66/1 -> A66/1
  "a45 "/1 -> A45/1
  a43/1(a34) -> A43/1
  a61/1 -> A61/1
  a21/1(a12) -> A21/1
  a22/1(a22) -> A22/1
  a25/1 -> A25/1
  a36/1 -> A36/1
  a33/1 -> A33/1
  a64/1 -> A64/1
  a32/1(a23) -> A32/1
  a46/1 -> A46/1
  "a65 "/1 -> A65/1
  a12/1(a12) -> A12/1
  "a15 "/1 -> A15/1
  a42/1 -> A42/1
  a26/1 -> A26/1
  a23/1(a23) -> A23/1
  a55/1 -> A55/1
  a34/1(a34) -> A34/1
  a51/1 -> A51/1
  a35/1(a35) -> A35/1
  a16/1 -> A16/1
  a56/1 -> A56/1

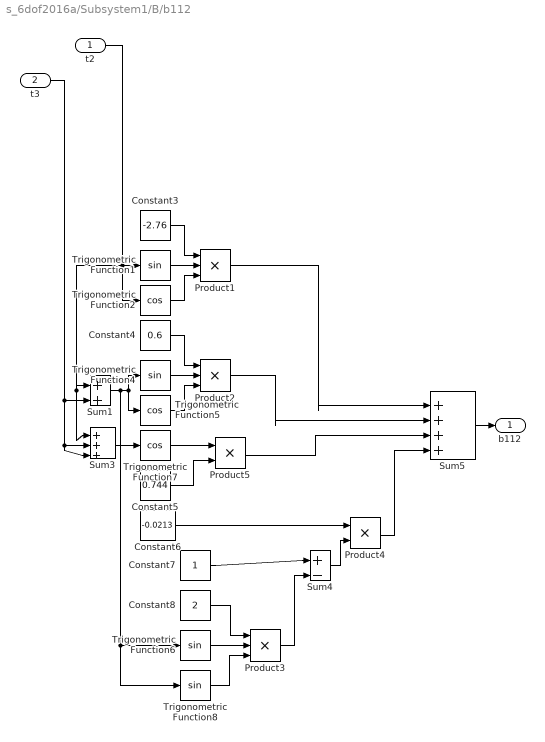
== system s_6dof2016a/Subsystem1/B/b112 ==
  t2 : Inport
  t3 : Inport  Port=2
  Constant3 : Constant  Value=-2.76
  Constant4 : Constant  Value=0.6
  Constant5 : Constant  Value=0.744
  Constant6 : Constant  Value=-0.0213
  Constant7 : Constant
  Constant8 : Constant  Value=2
  Product1 : Product  Inputs=3
  Product2 : Product  Inputs=3
  Product3 : Product  Inputs=3
  Product4 : Product
  Product5 : Product
  Sum1 : Sum  Inputs=|++
  Sum3 : Sum  Inputs=|+++
  Sum4 : Sum  Inputs=|+-
  Sum5 : Sum  Inputs=|++++
  Trigonometric Function{1,4,6,8} (4 alike) : Trigonometry
  Trigonometric Function2 : Trigonometry  Operator=cos
  Trigonometric Function5 : Trigonometry  Operator=cos
  Trigonometric Function7 : Trigonometry  Operator=cos
  b112 : Outport
  wires:
  t2/1 -> Sum3/1, Sum1/1, Trigonometric Function1/1, Trigonometric Function2/1
  Trigonometric Function1/1 -> Product1/2
  Trigonometric Function8/1 -> Product3/3
  t3/1 -> Sum3/3, Sum3/2, Sum1/2
  Constant5/1 -> Product5/2
  Sum5/1 -> b112/1
  Product3/1 -> Sum4/2
  Constant3/1 -> Product1/1
  Sum1/1 -> Trigonometric Function8/1, Trigonometric Function6/1, Trigonometric Function5/1, Trigonometric Function4/1
  Constant6/1 -> Product4/1
  Constant8/1 -> Product3/1
  Trigonometric Function7/1 -> Product5/1
  Constant4/1 -> Product2/1
  Constant7/1 -> Sum4/1
  Trigonometric Function5/1 -> Product2/3
  Product4/1 -> Sum5/4
  Product2/1 -> Sum5/2
  Trigonometric Function2/1 -> Product1/3
  Trigonometric Function6/1 -> Product3/2
  Trigonometric Function4/1 -> Product2/2
  Sum3/1 -> Trigonometric Function7/1
  Product1/1 -> Sum5/1
  Sum4/1 -> Product4/2
  Product5/1 -> Sum5/3

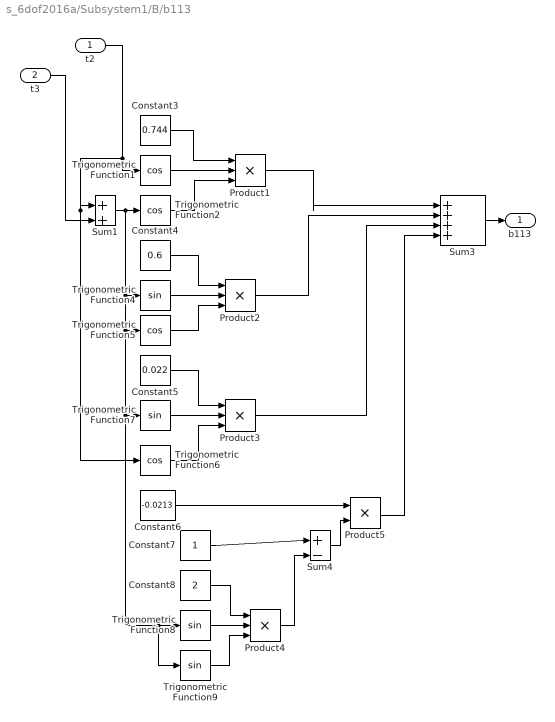
== system s_6dof2016a/Subsystem1/B/b113 ==
  t2 : Inport
  t3 : Inport  Port=2
  Constant3 : Constant  Value=0.744
  Constant4 : Constant  Value=0.6
  Constant5 : Constant  Value=0.022
  Constant6 : Constant  Value=-0.0213
  Constant7 : Constant
  Constant8 : Constant  Value=2
  Product{1..4} (4 alike) : Product  Inputs=3
  Product5 : Product
  Sum1 : Sum  Inputs=|++
  Sum3 : Sum  Inputs=|++++
  Sum4 : Sum  Inputs=|+-
  Trigonometric Function{1..2,5..6} (4 alike) : Trigonometry  Operator=cos
  Trigonometric Function{4,7..9} (4 alike) : Trigonometry
  b113 : Outport
  wires:
  Product2/1 -> Sum3/2
  t2/1 -> Trigonometric Function6/1, Sum1/1, Trigonometric Function1/1
  Trigonometric Function5/1 -> Product2/3
  Trigonometric Function1/1 -> Product1/2
  Constant3/1 -> Product1/1
  t3/1 -> Sum1/2
  Constant4/1 -> Product2/1
  Sum1/1 -> Trigonometric Function9/1, Trigonometric Function8/1, Trigonometric Function7/1, Trigonometric Function5/1, Trigonometric Function4/1, Trigonometric Function2/1
  Product3/1 -> Sum3/3
  Trigonometric Function9/1 -> Product4/3
  Constant6/1 -> Product5/1
  Trigonometric Function2/1 -> Product1/3
  Sum4/1 -> Product5/2
  Trigonometric Function8/1 -> Product4/2
  Sum3/1 -> b113/1
  Trigonometric Function7/1 -> Product3/2
  Constant8/1 -> Product4/1
  Constant7/1 -> Sum4/1
  Product4/1 -> Sum4/2
  Product5/1 -> Sum3/4
  Product1/1 -> Sum3/1
  Trigonometric Function4/1 -> Product2/2
  Trigonometric Function6/1 -> Product3/3
  Constant5/1 -> Product3/1

== system s_6dof2016a/Subsystem1/B/b114 ==
  t4 : Inport
  t5 : Inport  Port=2
  t2 : Inport  Port=3
  t3 : Inport  Port=4
  Constant3 : Constant  Value=-0.0025
  Constant4 : Constant  Value=0.00086
  Constant5 : Constant  Value=-0.00248
  Product1 : Product  Inputs=5
  Product2 : Product  Inputs=3
  Product3 : Product  Inputs=5
  Sum1 : Sum  Inputs=|++
  Sum3 : Sum  Inputs=|+++
  Trigonometric Function{1..2,4,7,10..11} (6 alike) : Trigonometry
  Trigonometric Function{5..6,8..9} (4 alike) : Trigonometry  Operator=cos
  b114 : Outport
  wires:
  t2/1 -> Sum1/1, Trigonometric Function9/1
  Trigonometric Function1/1 -> Product1/2
  t4/1 -> Trigonometric Function11/1, Trigonometric Function6/1, Trigonometric Function2/1
  Product1/1 -> Sum3/1
  Trigonometric Function11/1 -> Product3/4
  Trigonometric Function4/1 -> Product1/5
  Constant3/1 -> Product1/1
  t5/1 -> Trigonometric Function10/1, Trigonometric Function7/1, Trigonometric Function4/1
  Trigonometric Function10/1 -> Product3/5
  Trigonometric Function5/1 -> Product1/3
  Sum1/1 -> Trigonometric Function8/1, Trigonometric Function5/1, Trigonometric Function1/1
  Trigonometric Function8/1 -> Product3/2
  Trigonometric Function2/1 -> Product1/4
  Trigonometric Function9/1 -> Product3/3
  Constant5/1 -> Product3/1
  Trigonometric Function7/1 -> Product2/3
  Product3/1 -> Sum3/3
  Product2/1 -> Sum3/2
  Constant4/1 -> Product2/1
  Trigonometric Function6/1 -> Product2/2
  t3/1 -> Sum1/2
  Sum3/1 -> b114/1

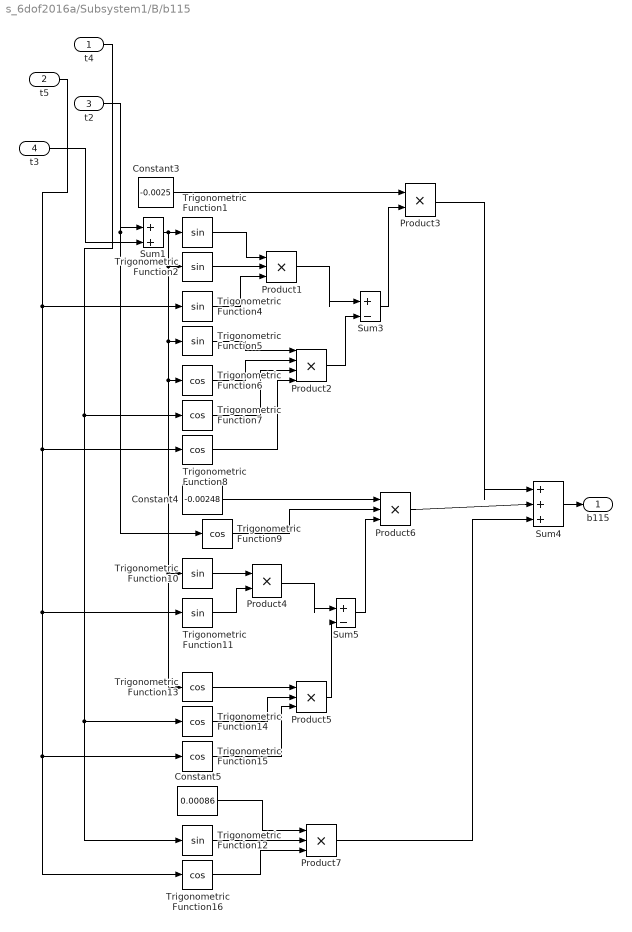
== system s_6dof2016a/Subsystem1/B/b115 ==
  t4 : Inport
  t5 : Inport  Port=2
  t2 : Inport  Port=3
  t3 : Inport  Port=4
  Constant3 : Constant  Value=-0.0025
  Constant4 : Constant  Value=-0.00248
  Constant5 : Constant  Value=0.00086
  Product{1,5..7} (4 alike) : Product  Inputs=3
  Product2 : Product  Inputs=4
  Product3 : Product
  Product4 : Product
  Sum1 : Sum  Inputs=|++
  Sum3 : Sum  Inputs=|+-
  Sum4 : Sum  Inputs=|+++
  Sum5 : Sum  Inputs=|+-
  Trigonometric Function{1..2,4..5,10..12} (7 alike) : Trigonometry
  Trigonometric Function{6..9,13..16} (8 alike) : Trigonometry  Operator=cos
  b115 : Outport
  wires:
  Trigonometric Function2/1 -> Product1/2
  Sum1/1 -> Trigonometric Function13/1, Trigonometric Function10/1, Trigonometric Function6/1, Trigonometric Function5/1, Trigonometric Function2/1, Trigonometric Function1/1
  Sum3/1 -> Product3/2
  Trigonometric Function16/1 -> Product7/3
  Trigonometric Function5/1 -> Product2/1
  Trigonometric Function4/1 -> Product1/3
  t4/1 -> Trigonometric Function12/1, Trigonometric Function14/1, Trigonometric Function7/1
  Product1/1 -> Sum3/1
  Product2/1 -> Sum3/2
  t5/1 -> Trigonometric Function16/1, Trigonometric Function15/1, Trigonometric Function11/1, Trigonometric Function8/1, Trigonometric Function4/1
  Trigonometric Function12/1 -> Product7/2
  Trigonometric Function6/1 -> Product2/2
  Trigonometric Function14/1 -> Product5/2
  t3/1 -> Sum1/2
  Product3/1 -> Sum4/1
  Product4/1 -> Sum5/1
  Trigonometric Function15/1 -> Product5/3
  Trigonometric Function10/1 -> Product4/1
  Trigonometric Function8/1 -> Product2/4
  Product6/1 -> Sum4/2
  Product7/1 -> Sum4/3
  Trigonometric Function7/1 -> Product2/3
  t2/1 -> Trigonometric Function9/1, Sum1/1
  Constant5/1 -> Product7/1
  Trigonometric Function1/1 -> Product1/1
  Sum5/1 -> Product6/3
  Trigonometric Function9/1 -> Product6/2
  Constant3/1 -> Product3/1
  Trigonometric Function11/1 -> Product4/2
  Constant4/1 -> Product6/1
  Product5/1 -> Sum5/2
  Trigonometric Function13/1 -> Product5/1
  Sum4/1 -> b115/1

== system s_6dof2016a/Subsystem1/B/b123 ==
  t2 : Inport
  "t3 " : Inport  Port=2
  Product1 : Product
  Product2 : Product
  Sum2 : Sum  Inputs=|++
  Sum3 : Sum  Inputs=|++
  Trigonometric Function : Trigonometry
  Trigonometric Function1 : Trigonometry  Operator=cos
  b1 : Constant  Value=0.267
  b2 : Constant  Value=-0.00758
  b123 : Outport
  wires:
  Trigonometric Function/1 -> Product2/2
  Product1/1 -> Sum3/2
  Sum3/1 -> b123/1
  Trigonometric Function1/1 -> Product1/2
  Sum2/1 -> Trigonometric Function1/1, Trigonometric Function/1
  b1/1 -> Product2/1
  Product2/1 -> Sum3/1
  b2/1 -> Product1/1
  "t3 "/1 -> Sum2/2
  t2/1 -> Sum2/1

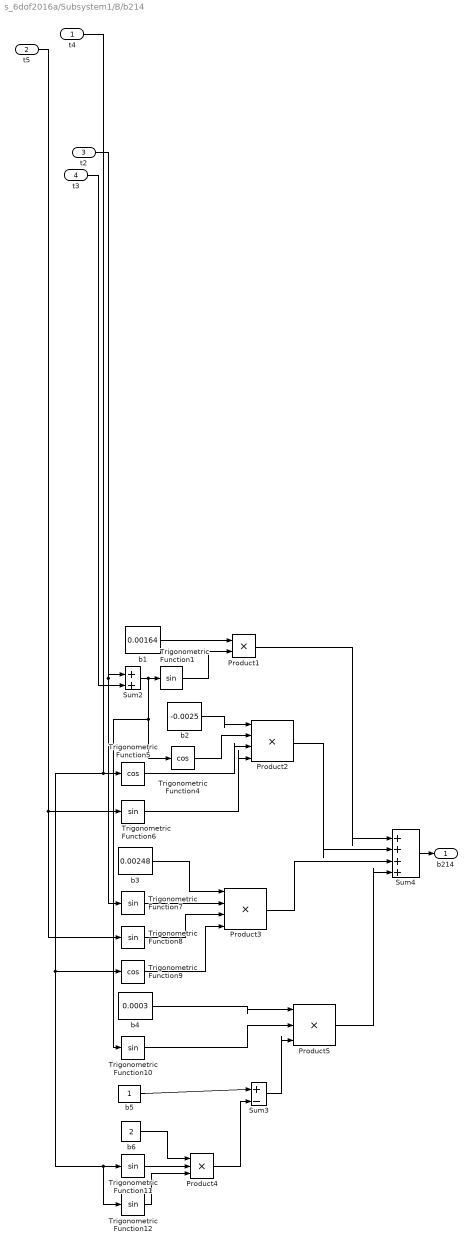
== system s_6dof2016a/Subsystem1/B/b214 ==
  t4 : Inport
  t5 : Inport  Port=2
  t2 : Inport  Port=3
  t3 : Inport  Port=4
  Product1 : Product
  Product2 : Product  Inputs=4
  Product3 : Product  Inputs=4
  Product4 : Product  Inputs=3
  Product5 : Product  Inputs=3
  Sum2 : Sum  Inputs=|++
  Sum3 : Sum  Inputs=|+-
  Sum4 : Sum  Inputs=|++++
  Trigonometric Function{1,6..8,10..12} (7 alike) : Trigonometry
  Trigonometric Function4 : Trigonometry  Operator=cos
  Trigonometric Function5 : Trigonometry  Operator=cos
  Trigonometric Function9 : Trigonometry  Operator=cos
  b1 : Constant  Value=0.00164
  b2 : Constant  Value=-0.0025
  b3 : Constant  Value=0.00248
  b4 : Constant  Value=0.0003
  b5 : Constant
  b6 : Constant  Value=2
  b214 : Outport
  wires:
  Sum2/1 -> Trigonometric Function10/1, Trigonometric Function4/1, Trigonometric Function1/1
  Trigonometric Function5/1 -> Product2/3
  Trigonometric Function1/1 -> Product1/2
  Trigonometric Function6/1 -> Product2/4
  Trigonometric Function10/1 -> Product5/2
  t2/1 -> Trigonometric Function7/1, Sum2/1
  t5/1 -> Trigonometric Function8/1, Trigonometric Function6/1
  b1/1 -> Product1/1
  Trigonometric Function4/1 -> Product2/2
  b6/1 -> Product4/1
  t4/1 -> Trigonometric Function12/1, Trigonometric Function11/1, Trigonometric Function9/1, Trigonometric Function5/1
  Product2/1 -> Sum4/2
  b2/1 -> Product2/1
  b5/1 -> Sum3/1
  Trigonometric Function11/1 -> Product4/2
  Trigonometric Function9/1 -> Product3/4
  Sum3/1 -> Product5/3
  b3/1 -> Product3/1
  Trigonometric Function7/1 -> Product3/2
  Trigonometric Function12/1 -> Product4/3
  b4/1 -> Product5/1
  Trigonometric Function8/1 -> Product3/3
  Product1/1 -> Sum4/1
  Product3/1 -> Sum4/3
  Product4/1 -> Sum3/2
  Sum4/1 -> b214/1
  Product5/1 -> Sum4/4
  t3/1 -> Sum2/2

== system s_6dof2016a/Subsystem1/B/b215 ==
  t4 : Inport
  t5 : Inport  Port=2
  t2 : Inport  Port=3
  t3 : Inport  Port=4
  Product1 : Product  Inputs=4
  Product2 : Product  Inputs=4
  Product3 : Product  Inputs=3
  Sum2 : Sum  Inputs=|++
  Sum3 : Sum  Inputs=|+++
  Trigonometric Function{1,4,8..9} (4 alike) : Trigonometry  Operator=cos
  Trigonometric Function{5..7,10} (4 alike) : Trigonometry
  b1 : Constant  Value=-0.0025
  b2 : Constant  Value=0.00248
  b3 : Constant  Value=-0.000642
  b215 : Outport
  wires:
  t4/1 -> Trigonometric Function10/1, Trigonometric Function7/1, Trigonometric Function5/1
  Trigonometric Function7/1 -> Product2/3
  Trigonometric Function1/1 -> Product1/2
  Trigonometric Function4/1 -> Product1/4
  Trigonometric Function8/1 -> Product2/4
  Trigonometric Function6/1 -> Product2/2
  b2/1 -> Product2/1
  t5/1 -> Trigonometric Function8/1, Trigonometric Function4/1
  t2/1 -> Trigonometric Function6/1, Sum2/1
  Trigonometric Function5/1 -> Product1/3
  Product2/1 -> Sum3/2
  Sum2/1 -> Trigonometric Function9/1, Trigonometric Function1/1
  Product3/1 -> Sum3/3
  Product1/1 -> Sum3/1
  Trigonometric Function9/1 -> Product3/2
  b3/1 -> Product3/1
  Trigonometric Function10/1 -> Product3/3
  b1/1 -> Product1/1
  t3/1 -> Sum2/2
  Sum3/1 -> b215/1

== system s_6dof2016a/Subsystem1/B/b223 ==
  t3 : Inport
  Product1 : Product
  Product2 : Product
  Sum2 : Sum  Inputs=|++
  Trigonometric Function1 : Trigonometry
  Trigonometric Function4 : Trigonometry  Operator=cos
  b1 : Constant  Value=0.022
  b2 : Constant  Value=0.744
  b223 : Outport
  wires:
  Sum2/1 -> b223/1
  b1/1 -> Product1/1
  b2/1 -> Product2/1
  Product2/1 -> Sum2/2
  t3/1 -> Trigonometric Function4/1, Trigonometric Function1/1
  Product1/1 -> Sum2/1
  Trigonometric Function4/1 -> Product2/2
  Trigonometric Function1/1 -> Product1/2

== system s_6dof2016a/Subsystem1/B/b224 ==
  t4 : Inport
  t5 : Inport  Port=2
  t3 : Inport  Port=3
  Product1 : Product  Inputs=4
  Trigonometric Function1 : Trigonometry  Operator=cos
  Trigonometric Function4 : Trigonometry
  Trigonometric Function5 : Trigonometry
  b1 : Constant  Value=-0.00248
  b224 : Outport
  wires:
  Trigonometric Function1/1 -> Product1/2
  Trigonometric Function5/1 -> Product1/4
  t5/1 -> Trigonometric Function5/1
  Trigonometric Function4/1 -> Product1/3
  b1/1 -> Product1/1
  Product1/1 -> b224/1
  t4/1 -> Trigonometric Function4/1
  t3/1 -> Trigonometric Function1/1

== system s_6dof2016a/Subsystem1/B/b225 ==
  t4 : Inport
  t5 : Inport  Port=2
  t3 : Inport  Port=3
  Constant3 : Constant  Value=-0.0025
  Constant4 : Constant  Value=0.00248
  Product1 : Product
  Product2 : Product  Inputs=3
  Product3 : Product
  Product4 : Product
  Sum2 : Sum  Inputs=|+-
  Sum3 : Sum  Inputs=|++
  Trigonometric Function1 : Trigonometry
  Trigonometric Function4 : Trigonometry  Operator=cos
  Trigonometric Function5 : Trigonometry  Operator=cos
  Trigonometric Function6 : Trigonometry  Operator=cos
  Trigonometric Function7 : Trigonometry
  Trigonometric Function8 : Trigonometry
  b225 : Outport
  wires:
  Sum2/1 -> Product4/2
  t5/1 -> Trigonometric Function8/1, Trigonometric Function6/1, Trigonometric Function1/1
  Trigonometric Function8/1 -> Product3/2
  Constant4/1 -> Product4/1
  Trigonometric Function6/1 -> Product2/3
  Product2/1 -> Sum2/1
  t3/1 -> Trigonometric Function7/1, Trigonometric Function4/1
  Trigonometric Function4/1 -> Product2/1
  Product1/1 -> Sum3/1
  Product4/1 -> Sum3/2
  Constant3/1 -> Product1/1
  Trigonometric Function7/1 -> Product3/1
  Trigonometric Function1/1 -> Product1/2
  Product3/1 -> Sum2/2
  Trigonometric Function5/1 -> Product2/2
  Sum3/1 -> b225/1
  t4/1 -> Trigonometric Function5/1

== system s_6dof2016a/Subsystem1/B/b234 ==
  t4 : Inport
  t5 : Inport  Port=2
  t3 : Inport  Port=3
  Product1 : Product  Inputs=4
  Trigonometric Function1 : Trigonometry  Operator=cos
  Trigonometric Function4 : Trigonometry
  Trigonometric Function5 : Trigonometry
  b1 : Constant  Value=-0.00248
  b224 : Outport
  wires:
  t3/1 -> Trigonometric Function1/1
  t4/1 -> Trigonometric Function4/1
  Product1/1 -> b224/1
  b1/1 -> Product1/1
  Trigonometric Function4/1 -> Product1/3
  t5/1 -> Trigonometric Function5/1
  Trigonometric Function5/1 -> Product1/4
  Trigonometric Function1/1 -> Product1/2

== system s_6dof2016a/Subsystem1/B/b235 ==
  t4 : Inport
  t5 : Inport  Port=2
  t3 : Inport  Port=3
  Constant3 : Constant  Value=-0.0025
  Constant4 : Constant  Value=0.00248
  Product1 : Product
  Product2 : Product  Inputs=3
  Product3 : Product
  Product4 : Product
  Sum2 : Sum  Inputs=|+-
  Sum3 : Sum  Inputs=|++
  Trigonometric Function1 : Trigonometry
  Trigonometric Function4 : Trigonometry  Operator=cos
  Trigonometric Function5 : Trigonometry  Operator=cos
  Trigonometric Function6 : Trigonometry  Operator=cos
  Trigonometric Function7 : Trigonometry
  Trigonometric Function8 : Trigonometry
  b225 : Outport
  wires:
  t4/1 -> Trigonometric Function5/1
  Sum3/1 -> b225/1
  Trigonometric Function5/1 -> Product2/2
  Product3/1 -> Sum2/2
  Trigonometric Function1/1 -> Product1/2
  Trigonometric Function7/1 -> Product3/1
  Constant3/1 -> Product1/1
  Product4/1 -> Sum3/2
  Product1/1 -> Sum3/1
  Trigonometric Function4/1 -> Product2/1
  t3/1 -> Trigonometric Function4/1, Trigonometric Function7/1
  Product2/1 -> Sum2/1
  Trigonometric Function6/1 -> Product2/3
  Constant4/1 -> Product4/1
  Trigonometric Function8/1 -> Product3/2
  t5/1 -> Trigonometric Function1/1, Trigonometric Function6/1, Trigonometric Function8/1
  Sum2/1 -> Product4/2

== system s_6dof2016a/Subsystem1/B/b314 ==
  t2 : Inport
  t4 : Inport  Port=2
  t5 : Inport  Port=3
  t3 : Inport  Port=4
  Constant3 : Constant  Value=0.00164
  Constant4 : Constant  Value=0.0003
  Constant5 : Constant  Value=2
  Constant6 : Constant
  Product1 : Product  Inputs=4
  Product2 : Product
  Product3 : Product  Inputs=3
  Product4 : Product  Inputs=3
  Sum2 : Sum  Inputs=|++
  Sum3 : Sum  Inputs=|+-
  Sum4 : Sum  Inputs=|+++
  Trigonometric Function1 : Trigonometry  Operator=cos
  Trigonometric Function4 : Trigonometry  Operator=cos
  Trigonometric Function{5..9} (5 alike) : Trigonometry
  b1 : Constant  Value=-0.0025
  b314 : Outport
  wires:
  t5/1 -> Trigonometric Function5/1
  Sum4/1 -> b314/1
  Sum2/1 -> Trigonometric Function7/1, Trigonometric Function6/1, Trigonometric Function1/1
  Product1/1 -> Sum4/1
  Constant5/1 -> Product3/1
  b1/1 -> Product1/1
  Product2/1 -> Sum4/2
  Trigonometric Function7/1 -> Product4/2
  Trigonometric Function9/1 -> Product3/3
  t4/1 -> Trigonometric Function4/1, Trigonometric Function9/1, Trigonometric Function8/1
  Sum3/1 -> Product4/3
  Trigonometric Function5/1 -> Product1/4
  Constant3/1 -> Product2/1
  Trigonometric Function6/1 -> Product2/2
  Trigonometric Function1/1 -> Product1/2
  Trigonometric Function4/1 -> Product1/3
  Product3/1 -> Sum3/2
  Product4/1 -> Sum4/3
  Constant6/1 -> Sum3/1
  Trigonometric Function8/1 -> Product3/2
  Constant4/1 -> Product4/1
  t3/1 -> Sum2/2
  t2/1 -> Sum2/1

== system s_6dof2016a/Subsystem1/B/b315 ==
  t2 : Inport
  t4 : Inport  Port=2
  t5 : Inport  Port=3
  t3 : Inport  Port=4
  Product1 : Product  Inputs=4
  Product2 : Product  Inputs=3
  Sum2 : Sum  Inputs=|++
  Sum3 : Sum  Inputs=|++
  Trigonometric Function1 : Trigonometry  Operator=cos
  Trigonometric Function4 : Trigonometry  Operator=cos
  Trigonometric Function5 : Trigonometry
  Trigonometric Function6 : Trigonometry  Operator=cos
  Trigonometric Function7 : Trigonometry
  b1 : Constant  Value=-0.0025
  b2 : Constant  Value=-0.000642
  b315 : Outport
  wires:
  Sum2/1 -> Trigonometric Function6/1, Trigonometric Function1/1
  Trigonometric Function4/1 -> Product1/4
  Trigonometric Function5/1 -> Product1/3
  Product1/1 -> Sum3/1
  Trigonometric Function1/1 -> Product1/2
  Product2/1 -> Sum3/2
  t3/1 -> Sum2/2
  Sum3/1 -> b315/1
  t4/1 -> Trigonometric Function7/1, Trigonometric Function5/1
  t2/1 -> Sum2/1
  Trigonometric Function7/1 -> Product2/3
  b2/1 -> Product2/1
  Trigonometric Function6/1 -> Product2/2
  b1/1 -> Product1/1
  t5/1 -> Trigonometric Function4/1

== system s_6dof2016a/Subsystem1/B/b325 ==
  t5 : Inport
  Product1 : Product
  Trigonometric Function1 : Trigonometry
  b1 : Constant  Value=-0.0025
  b325 : Outport
  wires:
  Trigonometric Function1/1 -> Product1/2
  b1/1 -> Product1/1
  Product1/1 -> b325/1
  t5/1 -> Trigonometric Function1/1

== system s_6dof2016a/Subsystem1/B/b335 ==
  t5 : Inport
  Product1 : Product
  Trigonometric Function1 : Trigonometry
  b1 : Constant  Value=-0.0025
  b325 : Outport
  wires:
  t5/1 -> Trigonometric Function1/1
  Product1/1 -> b325/1
  b1/1 -> Product1/1
  Trigonometric Function1/1 -> Product1/2

== system s_6dof2016a/Subsystem1/B/b345 ==
  t4 : Inport
  t5 : Inport  Port=2
  Product1 : Product  Inputs=3
  Trigonometric Function1 : Trigonometry
  Trigonometric Function4 : Trigonometry  Operator=cos
  b1 : Constant  Value=-0.0025
  b345 : Outport
  wires:
  b1/1 -> Product1/1
  Trigonometric Function4/1 -> Product1/3
  t5/1 -> Trigonometric Function4/1
  t4/1 -> Trigonometric Function1/1
  Trigonometric Function1/1 -> Product1/2
  Product1/1 -> b345/1

== system s_6dof2016a/Subsystem1/B/b412 ==
  t2 : Inport
  t3 : Inport  Port=2
  t4 : Inport  Port=3
  t5 : Inport  Port=4
  Product : Product
  b1 : Subsystem
  b2 : Constant  Value=-1
  b412 : Outport
  wires:
  t5/1 -> b1/2(t5)
  b2/1 -> Product/2
  Product/1 -> b412/1
  b1/1(b214) -> Product/1
  t2/1 -> b1/3(t2)
  t4/1 -> b1/1(t4)
  t3/1 -> b1/4(t3)

== system s_6dof2016a/Subsystem1/B/b413 ==
  In1 : Inport
  In2 : Inport  Port=2
  In3 : Inport  Port=3
  In4 : Inport  Port=4
  Constant : Constant  Value=-1
  Product : Product
  b1 : Subsystem
  b413 : Outport
  wires:
  b1/1(b314) -> Product/1
  In1/1 -> b1/1(t2)
  In3/1 -> b1/3(t5)
  Constant/1 -> Product/2
  In2/1 -> b1/2(t4)
  In4/1 -> b1/4(t3)
  Product/1 -> b413/1

== system s_6dof2016a/Subsystem1/B/b415 ==
  t2 : Inport
  t3 : Inport  Port=2
  t4 : Inport  Port=3
  Constant3 : Constant  Value=-0.000642
  Product1 : Product  Inputs=3
  Sum2 : Sum  Inputs=|++
  Trigonometric Function1 : Trigonometry  Operator=cos
  Trigonometric Function4 : Trigonometry
  b415 : Outport
  wires:
  Sum2/1 -> Trigonometric Function4/1
  Constant3/1 -> Product1/1
  t2/1 -> Sum2/1
  Product1/1 -> b415/1
  t3/1 -> Sum2/2
  Trigonometric Function1/1 -> Product1/3
  t4/1 -> Trigonometric Function1/1
  Trigonometric Function4/1 -> Product1/2

== system s_6dof2016a/Subsystem1/B/b425 ==
  t4 : Inport
  Product1 : Product
  Trigonometric Function1 : Trigonometry
  b1 : Constant  Value=0.000642
  b425 : Outport
  wires:
  Trigonometric Function1/1 -> Product1/2
  b1/1 -> Product1/1
  t4/1 -> Trigonometric Function1/1
  Product1/1 -> b425/1

== system s_6dof2016a/Subsystem1/B/b435 ==
  t4 : Inport
  Product1 : Product
  Trigonometric Function1 : Trigonometry
  b1 : Constant  Value=0.000642
  b425 : Outport
  wires:
  Trigonometric Function1/1 -> Product1/2
  b1/1 -> Product1/1
  t4/1 -> Trigonometric Function1/1
  Product1/1 -> b425/1

== system s_6dof2016a/Subsystem1/B/b512 ==
  t5 : Inport
  t2 : Inport  Port=2
  t3 : Inport  Port=3
  t4 : Inport  Port=4
  Constant3 : Constant  Value=-1
  Product1 : Product
  b1 : Subsystem
  b512 : Outport
  wires:
  t3/1 -> b1/4(t3)
  b1/1(b215) -> Product1/1
  t4/1 -> b1/1(t4)
  Constant3/1 -> Product1/2
  Product1/1 -> b512/1
  t2/1 -> b1/3(t2)
  t5/1 -> b1/2(t5)
